simulink model "Hybrid2_article_SVC_stage1"  (R2025a)
settings: Solver=FixedStepAuto  StartTime=0.0  StopTime=0.2  FixedStep=Ts  RelTol=1e-3
undefined symbols (not defined in the file or in its folder): closedLoop, controller, D1, D11, Delta, DiscIntNeverNeededParam, find_system, grid, level, protection, sensor, solarPanel, solarPlant, Ts
libraries: powerlib_extras x38, nesl_utility x29, spsSampleandHoldLib x24, spsThyristorLib x24, spsSeriesRLCBranchLib x23, simulink x22, fl_lib x18, ee_lib x12, spsEdgeDetectorLib x12, spsParallelRLCBranchLib x10, spsThreePhaseVIMeasurementLib x9, simulink_extras x8
(part 5 of 8)

== system Hybrid2_article_SVC_stage1/Power Circuit/Power Circuit/Average ==
  note: Resistance is added for simulation purpose, as the solver need to resolve absolute voltage values
  m : Inport
  TripSig : Inport  Port=2
  Average-Value Voltage Source Converter : ee_lib/Semiconductors & Converters/Converters/Average-Value Voltage Source Converter (Three-Phase)  port_option=ee.enum.threePhasePort.composite  frequency_option=ee.enum.converters.frequency.variable  input_option=ee.enum.converters.inputOption.ModWave  FRated=60 Hz  losses_parameterization=ee.enum.converters.losses.fixed  Pfixed=1 W  ks=0.01  kc1=1.7 V  kc2=0.01 Ohm  Ploss_vect=[100, 800, 1870, 3250, 4900] W  Irms_vect=[10, 100, 200, 300, 400] A  Vdc_nom=300 V  thermal_mass=30000 J/K  temperature_specify=off  temperature_priority=High  temperature=298.15 K  temperature_nominal_specify=off  temperature_nominal_value=1  temperature_nominal_unit=K
      settings: InternalSimscapePortConfiguration="{\"Bottom\":[],\"Left\":[{\"id\":\"ModWave\",\"label\":\"ModWave\",\"type\":\"input\"},{\"id\":\"N\",\"label\":\"~\",\"type\":\"foundation.electrical.three_phase\"}],\"Right\":[{\"id\":\"p\",\"label\":\"+\",\"type\":\"foundation.electrical.electrical\"},{\"id\":\"n\",\"label\":\"-\",\"type\":\"foundation.electrical.electrical\"}],\"Top\":[]}"
  Electrical Reference : fl_lib/Electrical/Electrical Elements/Electrical Reference
  Open Circuit : fl_lib/Electrical/Electrical Elements/Open Circuit  v_specify=off  v_priority=None  v=0 V  v_nominal_specify=off  v_nominal_value=1  v_nominal_unit=V
  Resistor : fl_lib/Electrical/Electrical Elements/Resistor  R=1e6 Ohm  i_specify=off  i_priority=None  i=0 A  i_nominal_specify=off  i_nominal_value=1  i_nominal_unit=A  v_specify=off  v_priority=None  v=0 V  v_nominal_specify=off  v_nominal_value=1  v_nominal_unit=V
  Simulink-PS Converter6 : nesl_utility/Simulink-PS Converter  PhysicalDomain=network_engine_domain  SubClassName=ps_input  LeftPortType=input  RightPortType=output  PseudoPeriodic=off  Frequencies=[]  NoiseDistribution=none  NoiseParameters=[]  Unit=1  AffineConversion=off  FilteringAndDerivatives=provide  SimscapeFilterOrder=1  InputFilterTimeConstant=0.001  UdotUserProvided=0
  Terminator : Terminator
  + : PMIOPort  Side=Left
  - : PMIOPort  Port=2  Side=Left
  ABC : PMIOPort  Port=3  Side=Right
  O : PMIOPort  Port=4  Side=Left
  wires:
  TripSig/1 -> Terminator/1
  m/1 -> Simulink-PS Converter6/1
  connections:
  Average-Value Voltage Source Converter/LConn2 -- ABC/RConn1
  Average-Value Voltage Source Converter/LConn1 -- Simulink-PS Converter6/RConn1
  Average-Value Voltage Source Converter/RConn2 -- Resistor/LConn1 -- -/RConn1
  Average-Value Voltage Source Converter/RConn1 -- +/RConn1
  Open Circuit/LConn1 -- O/RConn1
  Resistor/RConn1 -- Electrical Reference/LConn1

== system Hybrid2_article_SVC_stage1/Power Circuit/Power Circuit/Three Level ==
  m : Inport
  TripSig : Inport  Port=2
  Gate : Subsystem
  Neutral point controller : slpidlib/PID Controller  Controller=P  Form=Parallel  TimeDomain=Discrete-time  UseExternalTs=off  SampleTime=-1  IntegratorMethod=Forward Euler  FilterMethod=Forward Euler  ControllerParametersSource=internal  P=0.001  I=80/2  UseKiTs=off  D=0  UseExternalDerivativeSource=off  N=100  UseFilter=on  TunerSelectOption=Transfer Function Based (PID Tuner App)  ZeroCross=off  InitialConditionSource=internal  InitialConditionForIntegrator=0  InitialConditionForFilter=0  DifferentiatorICPrevScaledInput=0  ExternalReset=none  TrackingMode=off  Kt=1  LimitOutput=on  SatLimitsSource=internal  UpperSaturationLimit=1  LowerSaturationLimit=-1  LinearizeAsGain=on  AntiWindupMode=back-calculation  Kb=1000  LimitIntegrator=off  UpperIntegratorSaturationLimit=inf  LowerIntegratorSaturationLimit=-inf  POutMin=[]  POutMax=[]  IOutMin=[]  IOutMax=[]  DOutMin=[]  DOutMax=[]  NOutMin=[]  NOutMax=[]  SumOutMin=[]  SumOutMax=[]  SaturationOutMin=[]  SaturationOutMax=[]  PParamMin=[]  PParamMax=[]  IParamMin=[]  IParamMax=[]  DParamMin=[]  DParamMax=[]  NParamMin=[]  NParamMax=[]  KbParamMin=[]  KbParamMax=[]  KtParamMin=[]  KtParamMax=[]  KbOutMin=[]  KbOutMax=[]  KtOutMin=[]  KtOutMax=[]  IntegratorOutMin=[]  IntegratorOutMax=[]  FilterOutMin=[]  FilterOutMax=[]  SumI1OutMin=[]  SumI1OutMax=[]  SumI2OutMin=[]  SumI2OutMax=[]  SumI3OutMin=[]  SumI3OutMax=[]  SumI4OutMin=[]  SumI4OutMax=[]  SumDOutMin=[]  SumDOutMax=[]  DifferentiatorOutMin=[]  DifferentiatorOutMax=[]  FilterDiffOutCoefMin=[]  FilterDiffOutCoefMax=[]  ReciprocalOutMin=[]  ReciprocalOutMax=[]  SumDenOutMin=[]  SumDenOutMax=[]  SumNumOutMin=[]  SumNumOutMax=[]  DivideOutMin=[]  DivideOutMax=[]  UdiffTsProdOutMin=[]  UdiffTsProdOutMax=[]  NTsProdOutMin=[]  NTsProdOutMax=[]  UintegralTsProdOutMin=[]  UintegralTsProdOutMax=[]  UngainTsProdOutMin=[]  UngainTsProdOutMax=[]  ClampingZeroOutDataTypeStr=Inherit: Inherit via back propagation  ClampingZeroOutMin=[]  ClampingZeroOutMax=[]  FilterDenConstantOutDataTypeStr=Inherit: Inherit via back propagation  FilterDenConstantOutMin=[]  FilterDenConstantOutMax=[]  PCopyOutDataTypeStr=Inherit: Inherit via back propagation  PCopyOutMin=[]  PCopyOutMax=[]  NCopyOutDataTypeStr=Inherit: Inherit via back propagation  NCopyOutMin=[]  NCopyOutMax=[]  IntegratorContinuousStateAttributes=''  IntegratorStateMustResolveToSignalObject=off  IntegratorRTWStateStorageClass=Auto  FilterContinuousStateAttributes=''  FilterStateMustResolveToSignalObject=off  FilterRTWStateStorageClass=Auto  ParallelPVariant=InternalParameters  IdealPVariant=Disabled  IVariant=Disabled  DVariant=Disabled  IntegratorVariant=Disabled  SatVariant=Enabled  AWVariant=Disabled  PCopyVariant=Disabled  TRVariant=Disabled  FdbkBlocksVariant=Forward  IdealPFdbkVariant=Disabled  SatFdbkVariant=Disabled  DerivativeFilterVariant=Disabled  NVariant=Disabled  NCopyVariant=Disabled_SignalSpec  FilterICVariant=Disabled  IntegratorICVariant=Disabled  ExternalResetVariant=Disabled  TRSumVariant=Passthrough  SumFdbkVariant=Disabled  SumVariant=Passthrough_P  TsampFilterVariant=InternalTs  TsampNgainVariant=Passthrough  TsampIntegralVariant=Disabled_SignalSpec  ExternalSaturationOutDataTypeStr=Inherit: Same as second input  DerivativeSourceVariant=Disabled  PreIntVariant=InternalPreInt
  "PWM Generator (Three-phase, Three-level)" : eePwmGeneratorThreeLevel/PWM Generator (Three-phase, Three-level)  CPWMMode=SPWM: sinusoidal PWM  fsw=solarPlant.switchFrequency  Ts=1/(10*solarPlant.switchFrequency)
      settings: SamplingMode=Natural
  Product : Product
  Product1 : Product
  Protection : Subsystem
  Sensing voltage Vc1 : Subsystem
      mask Display: disp('Vdc1')
  Sensing voltage Vc2 : Subsystem
      mask Display: disp('Vdc2')
  Step@1cycle : Step  Time=1/grid.frequency  SampleTime=1/(10*solarPlant.switchFrequency)
  Sum : Sum  Inputs=|+-
  Switch5 : Switch  Criteria=u2 > Threshold  Threshold=solarPlant.DCMPPTValue/2/2  SaturateOnIntegerOverflow=off  InputSameDT=off
  Terminator1 : Terminator
  Three-Level Converter (Three-Phase) : ee_lib/Semiconductors & Converters/Converters/Three-Level Converter (Three-Phase)  port_option=ee.enum.threePhasePort.composite  device_type=2  Vf=0.8 V  Ron=0.001 Ohm  Rds=0.001 Ohm  Goff=1e-6 1/Ohm  Vth=0.2 V  Vgt=1 V  Vgt_off=-1 V  Ih=1 A  K=0  diode_param=2  diode_Vf=0.8 V  diode_Ron=0.001 Ohm  diode_Goff=1e-5 1/Ohm  diode_C=50 nF  diode_iRM=-235 A  diode_iF=300 A  diode_idot=-50 A/us  diode_trr_param=1  diode_trr_factor=3  diode_trr=15 us  diode_Qrr=1500 s*uA  snubber_type=0  Cs=1e-7 F  Rs=0.1 Ohm
      settings: InternalSimscapePortConfiguration="{\"Bottom\":[],\"Left\":[{\"id\":\"G\",\"label\":\"G\",\"type\":\"foundation.electrical.twenty_four_phase\"},{\"id\":\"N\",\"label\":\"~\",\"type\":\"foundation.electrical.three_phase\"}],\"Right\":[{\"id\":\"p\",\"label\":\"+\",\"type\":\"foundation.electrical.electrical\"},{\"id\":\"z\",\"label\":\"0\",\"type\":\"foundation.electrical.electrical\"},{\"id\":\"n\",\"label\":\"-\",\"type\":\"foundation.electrical.electrical\"}],\"Top\":[]}"
  Zero-Order Hold1 : ZeroOrderHold  SampleTime=1/(10*solarPlant.switchFrequency)
  Zero-Order Hold2 : ZeroOrderHold  SampleTime=1/(5*solarPlant.switchFrequency)
  Zero-Order Hold3 : ZeroOrderHold  SampleTime=1/(5*solarPlant.switchFrequency)
  Zero-Order Hold4 : ZeroOrderHold  SampleTime=1/(10*solarPlant.switchFrequency)
  start MPPT Voltage : Constant  Value=solarPlant.DCMPPTValue/2
  + : PMIOPort  Side=Left
  - : PMIOPort  Port=2  Side=Left
  ABC : PMIOPort  Port=3  Side=Right
  O : PMIOPort  Port=4  Side=Left
  wires:
  Sum/1 -> Neutral point controller/1
  Switch5/1 -> Zero-Order Hold4/1, Product1/2
  m/1 -> Product1/1
  Zero-Order Hold2/1 -> Sum/1
  [Vpv] -> Switch5/2, Switch5/1
  Protection/1(PWM) -> Gate/1(g)
  Zero-Order Hold3/1 -> Sum/2
  "PWM Generator (Three-phase, Three-level)"/1 -> Protection/2(G)
  Zero-Order Hold1/1 -> "PWM Generator (Three-phase, Three-level)"/1
  Zero-Order Hold4/1 -> "PWM Generator (Three-phase, Three-level)"/2
  "PWM Generator (Three-phase, Three-level)"/2 -> Terminator1/1
  Product1/1 -> Zero-Order Hold1/1
  [Vdc1] -> Zero-Order Hold2/1
  start MPPT Voltage/1 -> Switch5/3
  TripSig/1 -> Protection/1(TripSig)
  Step@1cycle/1 -> Product/2
  [Vdc2] -> Zero-Order Hold3/1
  Neutral point controller/1 -> Product/1
  Product/1 -> "PWM Generator (Three-phase, Three-level)"/3
  connections:
  Three-Level Converter (Three-Phase)/RConn2 -- O/RConn1 -- Sensing voltage Vc2/LConn1 -- Sensing voltage Vc1/RConn1
  Three-Level Converter (Three-Phase)/RConn3 -- -/RConn1 -- Sensing voltage Vc2/RConn1
  Three-Level Converter (Three-Phase)/RConn1 -- +/RConn1 -- Sensing voltage Vc1/LConn1
  Three-Level Converter (Three-Phase)/LConn2 -- ABC/RConn1
  Gate/RConn1 -- Three-Level Converter (Three-Phase)/LConn1

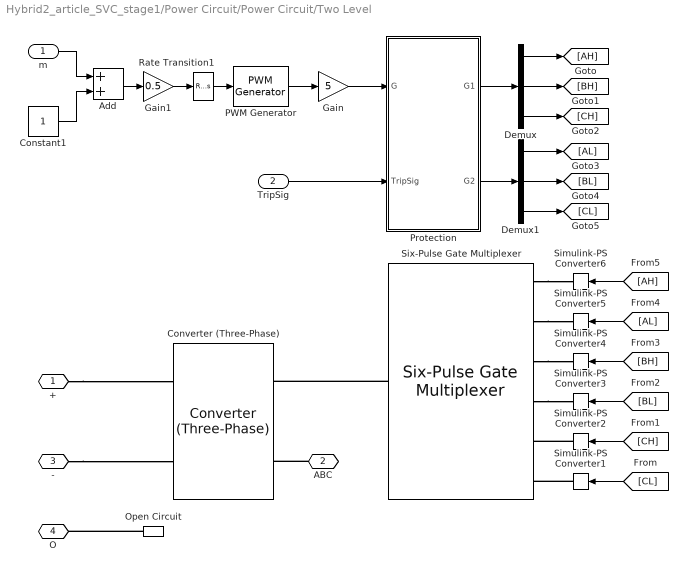
== system Hybrid2_article_SVC_stage1/Power Circuit/Power Circuit/Two Level ==
  m : Inport
  TripSig : Inport  Port=2
  Add : Sum
  Constant1 : Constant
  Converter (Three-Phase) : ee_lib/Semiconductors & Converters/Converters/Converter (Three-Phase)  port_option=ee.enum.threePhasePort.composite  fidelity_option=ee.enum.converters.fidelity.detailed  device_type=ee.enum.converters.switchingdevice.ideal  showThermalPort=false  K=0  Vth=0.5 V  Vgt=1 V  Vgt_off=-1 V  Ih=1 A  Vf=0.8 V  Ron=0.001 Ohm  Rds=0.001 Ohm  Goff=1e-6 1/Ohm  Eon_scalar=22.86e-3 J  Eoff_scalar=17.14e-3 J  Eoff_natural_commutation=10e-3 J  Voff=300 V  Iout_scalar=600 A  onCurrentMeasDelay=0 s  useCurrentFromPreviousCycle=false  useVoltageFromPreviousCycle=false  diode_param=ee.enum.converters.protectiondiode.nodynamics  diode_Vf=0.01 V  diode_Ron=0.0001 Ohm  diode_Goff=1e-5 1/Ohm  diode_C=50 nF  diode_iRM=-235 A  diode_iF=300 A  diode_idot=-50 A/us  diode_trr_param=ee.enum.converters.diodetrr.trr_factor  diode_trr_factor=3  diode_trr=15 us  diode_Qrr=1500 s*uA  diode_rec_loss_model=ee.enum.diode.reverseRecoveryModel.fixed  diode_ErecVal=0 J  diode_scaleWithIandV=false  diode_ErecMat=zeros(2, 3) J  diode_TjrecVec=[298.15, 398.15] K  diode_IfrecVec=[.1, 1, 10] A  diode_IrecVal=10 A  diode_VrecVal=10 V  diode_tFilter=1 / 1000 / 100 s  thermal_network_parameterization=ee.enum.thermalNetworkTopology.external  Rth=[.08, .5] K/W  Rth_Cauer=[.08, .1, .5] K/W  Rth_Foster=[.08, .14, .22, .16] K/W  thermal_mass_parameterization=ee.enum.thermalNetwork.timeconstant  thermal_mass=[.01, .5] J/K  thermal_mass_Cauer=[.01, .1, .5] J/K  thermal_mass_Foster=[.001, .005, .05, .5] J/K  thermal_time_constant=[.001, .2] s  thermal_time_constant_Cauer=[.001, .1, .2] s  thermal_time_constant_Foster=[7e-05, .0007, .01, .08] s  thermal_mass_initial_temperatures=[25, 25] degC  thermal_mass_initial_temperatures_Cauer=[25, 25, 25] degC  junction_thermal_mass=0.01 J/K  Tvec_initial_Foster=[25, 25, 25, 25] degC  snubber_type=ee.enum.converters.snubber.exclude  Cs=1e-7 F  Rs=0.1 Ohm  Vce_loss=[0, 150, 300] V
  Demux : Demux  Outputs=3
  Demux1 : Demux  Outputs=3
  Gain : Gain  Gain=5
  Gain1 : Gain  Gain=0.5
  Open Circuit : fl_lib/Electrical/Electrical Elements/Open Circuit  v_specify=off  v_priority=None  v=0 V  v_nominal_specify=off  v_nominal_value=1  v_nominal_unit=V
  PWM Generator : eePwmGenerator/PWM Generator  CarrCount=Up  Tper=1/solarPlant.switchFrequency  Tdelay=0  Ts=1/(10*solarPlant.switchFrequency)
  Protection : Subsystem
  Rate Transition1 : RateTransition  OutPortSampleTime=1/(10*solarPlant.switchFrequency)
  Simulink-PS Converter{1..6} (6 alike) : nesl_utility/Simulink-PS Converter  PhysicalDomain=network_engine_domain  SubClassName=ps_input  LeftPortType=input  RightPortType=output  PseudoPeriodic=off  Frequencies=[]  NoiseDistribution=none  NoiseParameters=[]  Unit=1  AffineConversion=off  FilteringAndDerivatives=provide  SimscapeFilterOrder=1  InputFilterTimeConstant=0.001  UdotUserProvided=0
  Six-Pulse Gate Multiplexer : ee_lib/Semiconductors & Converters/Converters/Six-Pulse Gate Multiplexer  port_option=ee.enum.controlport.ps
  + : PMIOPort  Side=Left
  ABC : PMIOPort  Port=2  Side=Right
  - : PMIOPort  Port=3  Side=Left
  O : PMIOPort  Port=4  Side=Left
  wires:
  Rate Transition1/1 -> PWM Generator/1
  [CL] -> Simulink-PS Converter1/1
  [AH] -> Simulink-PS Converter6/1
  Demux1/3 -> [CL]
  m/1 -> Add/1
  [CH] -> Simulink-PS Converter2/1
  Demux/2 -> [BH]
  Demux1/2 -> [BL]
  Demux/3 -> [CH]
  TripSig/1 -> Protection/2(TripSig)
  Demux1/1 -> [AL]
  [BH] -> Simulink-PS Converter4/1
  Protection/2(G2) -> Demux1/1
  Protection/1(G1) -> Demux/1
  PWM Generator/1 -> Gain/1
  [AL] -> Simulink-PS Converter5/1
  [BL] -> Simulink-PS Converter3/1
  Constant1/1 -> Add/2
  Gain/1 -> Protection/1(G)
  Add/1 -> Gain1/1
  Gain1/1 -> Rate Transition1/1
  Demux/1 -> [AH]
  connections:
  Open Circuit/LConn1 -- O/RConn1
  Simulink-PS Converter2/RConn1 -- Six-Pulse Gate Multiplexer/LConn5
  ABC/RConn1 -- Converter (Three-Phase)/LConn2
  Six-Pulse Gate Multiplexer/RConn1 -- Converter (Three-Phase)/LConn1
  Six-Pulse Gate Multiplexer/LConn2 -- Simulink-PS Converter5/RConn1
  +/RConn1 -- Converter (Three-Phase)/RConn1
  -/RConn1 -- Converter (Three-Phase)/RConn2
  Six-Pulse Gate Multiplexer/LConn4 -- Simulink-PS Converter3/RConn1
  Six-Pulse Gate Multiplexer/LConn3 -- Simulink-PS Converter4/RConn1
  Six-Pulse Gate Multiplexer/LConn1 -- Simulink-PS Converter6/RConn1
  Simulink-PS Converter1/RConn1 -- Six-Pulse Gate Multiplexer/LConn6

== system Hybrid2_article_SVC_stage1/SVC Controller1/Firing Unit/Firing Unit AB ==
  note: PLL
      | sync on
      | pos. peak
      | of input
  note: Generate firing
      | pulses for TSC3
  note: Generate firing
      | pulse for TCR +
  note: Generate firing
      | pulse for TCR -
  note: Generate firing
      | pulses for TSC2
  note: Generate firing
      | pulses for TSC1
  note: Generate square-wave lagging Input
      | voltage by 90 degrees and pulses (width of
      | one sample) for positive (Sync +)
      | and negative (Sync -) transition
  note: Compute number
      | of samples per cycle
  note: Input
      | voltage
  V : Inport  PortDimensions=1
  Alpha : Inport  Port=2  PortDimensions=1
  TSC1_On : Inport  Port=3  PortDimensions=1
  TSC2_On : Inport  Port=4  PortDimensions=1
  TSC3_On : Inport  Port=5  PortDimensions=1
  BL2 : Subsystem
  BL3 : Subsystem
  Correction for delay : Gain  Gain=Nstep*Ts*2*pi  SaturateOnIntegerOverflow=on  OutDataTypeStr=Inherit: Same as input  ParamDataTypeStr=Inherit: Same as input
  Logical Operator2 : Logic  Operator=NOT  Inputs=3
  "PLL sync on positive peak " : Subsystem  mask(Discrete 1-phase PLL){Par_Init=[PhaseInit FreqInit], ParK=[120 2800], Ts=Ts}
      mask prompts: Par_Init "Initial input:[ Phase(degrees)   Frequency(Hz) ]"; ParK "Regulator gains [ Kp  Ki ]"; Ts "Sample time:"
      mask help:
      | This Phase Locked Loop (PLL) system can be used  to synchronize on a variable frequency sinusoidal signal.
      |
      | Input 1: Normalized input signal V(pu)
      mask init:
      | Kp=ParK(1);
      | Ki=ParK(2);
      | Phase_Init=Par_Init(1);
      | Finit=Par_Init(2);
  Sum : Sum  InputSameDT=on  SaturateOnIntegerOverflow=on  OutDataTypeStr=Inherit: Same as first input
  TCR Pulse Generatorr : Subsystem
  TCR Pulse Generatorr1 : Subsystem  mask{Ts=Ts}
      mask prompts: Ts "Sample time:"
  TCS Pulse Generator : Subsystem
  TCS Pulse Generator1 : Subsystem
  TCS Pulse Generator2 : Subsystem
  Trigonometric Function6 : Trigonometry
  TCR + : Outport  VectorParamsAs1DForOutWhenUnconnected=off
  TCR - : Outport  Port=2  VectorParamsAs1DForOutWhenUnconnected=off
  TSC1 + : Outport  Port=3  VectorParamsAs1DForOutWhenUnconnected=off
  TSC1 - : Outport  Port=4  VectorParamsAs1DForOutWhenUnconnected=off
  TSC2 + : Outport  Port=5  VectorParamsAs1DForOutWhenUnconnected=off
  TSC2 - : Outport  Port=6  VectorParamsAs1DForOutWhenUnconnected=off
  TSC3 + : Outport  Port=7  VectorParamsAs1DForOutWhenUnconnected=off
  TSC3 - : Outport  Port=8  VectorParamsAs1DForOutWhenUnconnected=off
  wires:
  Logical Operator2/1 -> TCR Pulse Generatorr1/4(SqWave)
  TCR Pulse Generatorr/1(TCR +/-) -> TCR +/1
  BL3/1(SqWave) -> TCS Pulse Generator/1(SqWave), TCS Pulse Generator2/1(SqWave), TCS Pulse Generator1/1(SqWave), TCR Pulse Generatorr/4(SqWave), Logical Operator2/1
  TCS Pulse Generator2/2(TSC -) -> TSC3 -/1
  TCS Pulse Generator2/1(TSC +) -> TSC3 +/1
  TSC3_On/1 -> TCS Pulse Generator2/4(TSC_On)
  TCR Pulse Generatorr1/1(TCR +/-) -> TCR -/1
  TCS Pulse Generator/2(TSC -) -> TSC1 -/1
  TCS Pulse Generator/1(TSC +) -> TSC1 +/1
  BL3/2(Sync +) -> TCS Pulse Generator2/2(Sync +), TCS Pulse Generator1/2(Sync +), TCS Pulse Generator/2(Sync +), TCR Pulse Generatorr/3(Sync +/-)
  BL3/3(Sync -) -> TCS Pulse Generator/3(Sync -), TCS Pulse Generator2/3(Sync -), TCS Pulse Generator1/3(Sync -), TCR Pulse Generatorr1/3(Sync +/-)
  Alpha/1 -> TCR Pulse Generatorr/2(Alpha), TCR Pulse Generatorr1/2(Alpha)
  TSC1_On/1 -> TCS Pulse Generator/4(TSC_On)
  TCS Pulse Generator1/2(TSC -) -> TSC2 -/1
  TCS Pulse Generator1/1(TSC +) -> TSC2 +/1
  TSC2_On/1 -> TCS Pulse Generator1/4(TSC_On)
  BL2/1(Ns/c) -> TCR Pulse Generatorr/1(Ns/c), TCR Pulse Generatorr1/1(Ns/c)
  "PLL sync on positive peak "/2(wt) -> Sum/2
  Sum/1 -> Trigonometric Function6/1
  Trigonometric Function6/1 -> BL3/2(sin(wt))
  Correction for delay/1 -> Sum/1
  "PLL sync on positive peak "/1(Freq) -> BL2/1(Freq), BL3/1(Freq), Correction for delay/1
  V/1 -> "PLL sync on positive peak "/1(V(pu))

== system Hybrid2_article_SVC_stage1/SVC Controller1/Firing Unit/Firing Unit BC ==
  note: PLL
      | sync on
      | pos. peak
      | of input
  note: Generate firing
      | pulses for TSC3
  note: Generate firing
      | pulse for TCR +
  note: Generate firing
      | pulse for TCR -
  note: Generate firing
      | pulses for TSC2
  note: Generate firing
      | pulses for TSC1
  note: Generate square-wave lagging Input
      | voltage by 90 degrees and pulses (width of
      | one sample) for positive (Sync +)
      | and negative (Sync -) transition
  note: Compute number
      | of samples per cycle
  note: Input
      | voltage
  V : Inport  PortDimensions=1
  Alpha : Inport  Port=2  PortDimensions=1
  TSC1_On : Inport  Port=3  PortDimensions=1
  TSC2_On : Inport  Port=4  PortDimensions=1
  TSC3_On : Inport  Port=5  PortDimensions=1
  BL2 : Subsystem
  BL3 : Subsystem
  Correction for delay : Gain  Gain=Nstep*Ts*2*pi  SaturateOnIntegerOverflow=on  OutDataTypeStr=Inherit: Same as input  ParamDataTypeStr=Inherit: Same as input
  Logical Operator2 : Logic  Operator=NOT  Inputs=3
  "PLL sync on positive peak " : Subsystem  mask(Discrete 1-phase PLL){Par_Init=[PhaseInit FreqInit], ParK=[120 2800], Ts=Ts}
      mask prompts: Par_Init "Initial input:[ Phase(degrees)   Frequency(Hz) ]"; ParK "Regulator gains [ Kp  Ki ]"; Ts "Sample time:"
      mask help:
      | This Phase Locked Loop (PLL) system can be used  to synchronize on a variable frequency sinusoidal signal.
      |
      | Input 1: Normalized input signal V(pu)
      mask init:
      | Kp=ParK(1);
      | Ki=ParK(2);
      | Phase_Init=Par_Init(1);
      | Finit=Par_Init(2);
  Sum : Sum  InputSameDT=on  SaturateOnIntegerOverflow=on  OutDataTypeStr=Inherit: Same as first input
  TCR Pulse Generatorr : Subsystem  mask{Ts=Ts}
      mask prompts: Ts "Sample time:"
  TCR Pulse Generatorr1 : Subsystem  mask{Ts=Ts}
      mask prompts: Ts "Sample time:"
  TCS Pulse Generator : Subsystem
  TCS Pulse Generator1 : Subsystem
  TCS Pulse Generator2 : Subsystem
  Trigonometric Function6 : Trigonometry
  TCR + : Outport  VectorParamsAs1DForOutWhenUnconnected=off
  TCR - : Outport  Port=2  VectorParamsAs1DForOutWhenUnconnected=off
  TSC1 + : Outport  Port=3  VectorParamsAs1DForOutWhenUnconnected=off
  TSC1 - : Outport  Port=4  VectorParamsAs1DForOutWhenUnconnected=off
  TSC2 + : Outport  Port=5  VectorParamsAs1DForOutWhenUnconnected=off
  TSC2 - : Outport  Port=6  VectorParamsAs1DForOutWhenUnconnected=off
  TSC3 + : Outport  Port=7  VectorParamsAs1DForOutWhenUnconnected=off
  TSC3 - : Outport  Port=8  VectorParamsAs1DForOutWhenUnconnected=off
  wires:
  Logical Operator2/1 -> TCR Pulse Generatorr1/4(SqWave)
  TCR Pulse Generatorr/1(TCR +/-) -> TCR +/1
  BL3/1(SqWave) -> TCS Pulse Generator/1(SqWave), TCS Pulse Generator2/1(SqWave), TCS Pulse Generator1/1(SqWave), TCR Pulse Generatorr/4(SqWave), Logical Operator2/1
  TCS Pulse Generator2/2(TSC -) -> TSC3 -/1
  TCS Pulse Generator2/1(TSC +) -> TSC3 +/1
  TSC3_On/1 -> TCS Pulse Generator2/4(TSC_On)
  TCR Pulse Generatorr1/1(TCR +/-) -> TCR -/1
  TCS Pulse Generator/2(TSC -) -> TSC1 -/1
  TCS Pulse Generator/1(TSC +) -> TSC1 +/1
  BL3/2(Sync +) -> TCS Pulse Generator2/2(Sync +), TCS Pulse Generator1/2(Sync +), TCS Pulse Generator/2(Sync +), TCR Pulse Generatorr/3(Sync +/-)
  BL3/3(Sync -) -> TCS Pulse Generator/3(Sync -), TCS Pulse Generator2/3(Sync -), TCS Pulse Generator1/3(Sync -), TCR Pulse Generatorr1/3(Sync +/-)
  Alpha/1 -> TCR Pulse Generatorr/2(Alpha), TCR Pulse Generatorr1/2(Alpha)
  TSC1_On/1 -> TCS Pulse Generator/4(TSC_On)
  TCS Pulse Generator1/2(TSC -) -> TSC2 -/1
  TCS Pulse Generator1/1(TSC +) -> TSC2 +/1
  TSC2_On/1 -> TCS Pulse Generator1/4(TSC_On)
  BL2/1(Ns/c) -> TCR Pulse Generatorr/1(Ns/c), TCR Pulse Generatorr1/1(Ns/c)
  "PLL sync on positive peak "/2(wt) -> Sum/2
  Sum/1 -> Trigonometric Function6/1
  Trigonometric Function6/1 -> BL3/2(sin(wt))
  Correction for delay/1 -> Sum/1
  "PLL sync on positive peak "/1(Freq) -> BL2/1(Freq), BL3/1(Freq), Correction for delay/1
  V/1 -> "PLL sync on positive peak "/1(V(pu))

== system Hybrid2_article_SVC_stage1/SVC Controller1/Firing Unit/Firing Unit CA ==
  note: PLL
      | sync on
      | pos. peak
      | of input
  note: Generate firing
      | pulses for TSC3
  note: Generate firing
      | pulse for TCR +
  note: Generate firing
      | pulse for TCR -
  note: Generate firing
      | pulses for TSC2
  note: Generate firing
      | pulses for TSC1
  note: Generate square-wave lagging Input
      | voltage by 90 degrees and pulses (width of
      | one sample) for positive (Sync +)
      | and negative (Sync -) transition
  note: Compute number
      | of samples per cycle
  note: Input
      | voltage
  V : Inport  PortDimensions=1
  Alpha : Inport  Port=2  PortDimensions=1
  TSC1_On : Inport  Port=3  PortDimensions=1
  TSC2_On : Inport  Port=4  PortDimensions=1
  TSC3_On : Inport  Port=5  PortDimensions=1
  BL2 : Subsystem
  BL3 : Subsystem
  Correction for delay : Gain  Gain=Nstep*Ts*2*pi  SaturateOnIntegerOverflow=on  OutDataTypeStr=Inherit: Same as input  ParamDataTypeStr=Inherit: Same as input
  Logical Operator2 : Logic  Operator=NOT  Inputs=3
  "PLL sync on positive peak " : Subsystem  mask(Discrete 1-phase PLL){Par_Init=[PhaseInit FreqInit], ParK=[120 2800], Ts=Ts}
      mask prompts: Par_Init "Initial input:[ Phase(degrees)   Frequency(Hz) ]"; ParK "Regulator gains [ Kp  Ki ]"; Ts "Sample time:"
      mask help:
      | This Phase Locked Loop (PLL) system can be used  to synchronize on a variable frequency sinusoidal signal.
      |
      | Input 1: Normalized input signal V(pu)
      mask init:
      | Kp=ParK(1);
      | Ki=ParK(2);
      | Phase_Init=Par_Init(1);
      | Finit=Par_Init(2);
  Sum : Sum  InputSameDT=on  SaturateOnIntegerOverflow=on  OutDataTypeStr=Inherit: Same as first input
  TCR Pulse Generatorr : Subsystem  mask{Ts=Ts}
      mask prompts: Ts "Sample time:"
  TCR Pulse Generatorr1 : Subsystem  mask{Ts=Ts}
      mask prompts: Ts "Sample time:"
  TCS Pulse Generator : Subsystem
  TCS Pulse Generator1 : Subsystem
  TCS Pulse Generator2 : Subsystem
  Trigonometric Function6 : Trigonometry
  TCR + : Outport  VectorParamsAs1DForOutWhenUnconnected=off
  TCR - : Outport  Port=2  VectorParamsAs1DForOutWhenUnconnected=off
  TSC1 + : Outport  Port=3  VectorParamsAs1DForOutWhenUnconnected=off
  TSC1 - : Outport  Port=4  VectorParamsAs1DForOutWhenUnconnected=off
  TSC2 + : Outport  Port=5  VectorParamsAs1DForOutWhenUnconnected=off
  TSC2 - : Outport  Port=6  VectorParamsAs1DForOutWhenUnconnected=off
  TSC3 + : Outport  Port=7  VectorParamsAs1DForOutWhenUnconnected=off
  TSC3 - : Outport  Port=8  VectorParamsAs1DForOutWhenUnconnected=off
  wires:
  Logical Operator2/1 -> TCR Pulse Generatorr1/4(SqWave)
  TCR Pulse Generatorr/1(TCR +/-) -> TCR +/1
  BL3/1(SqWave) -> TCS Pulse Generator/1(SqWave), TCS Pulse Generator2/1(SqWave), TCS Pulse Generator1/1(SqWave), TCR Pulse Generatorr/4(SqWave), Logical Operator2/1
  TCS Pulse Generator2/2(TSC -) -> TSC3 -/1
  TCS Pulse Generator2/1(TSC +) -> TSC3 +/1
  TSC3_On/1 -> TCS Pulse Generator2/4(TSC_On)
  TCR Pulse Generatorr1/1(TCR +/-) -> TCR -/1
  TCS Pulse Generator/2(TSC -) -> TSC1 -/1
  TCS Pulse Generator/1(TSC +) -> TSC1 +/1
  BL3/2(Sync +) -> TCS Pulse Generator2/2(Sync +), TCS Pulse Generator1/2(Sync +), TCS Pulse Generator/2(Sync +), TCR Pulse Generatorr/3(Sync +/-)
  BL3/3(Sync -) -> TCS Pulse Generator/3(Sync -), TCS Pulse Generator2/3(Sync -), TCS Pulse Generator1/3(Sync -), TCR Pulse Generatorr1/3(Sync +/-)
  Alpha/1 -> TCR Pulse Generatorr/2(Alpha), TCR Pulse Generatorr1/2(Alpha)
  TSC1_On/1 -> TCS Pulse Generator/4(TSC_On)
  TCS Pulse Generator1/2(TSC -) -> TSC2 -/1
  TCS Pulse Generator1/1(TSC +) -> TSC2 +/1
  TSC2_On/1 -> TCS Pulse Generator1/4(TSC_On)
  BL2/1(Ns/c) -> TCR Pulse Generatorr/1(Ns/c), TCR Pulse Generatorr1/1(Ns/c)
  "PLL sync on positive peak "/2(wt) -> Sum/2
  Sum/1 -> Trigonometric Function6/1
  Trigonometric Function6/1 -> BL3/2(sin(wt))
  Correction for delay/1 -> Sum/1
  "PLL sync on positive peak "/1(Freq) -> BL2/1(Freq), BL3/1(Freq), Correction for delay/1
  V/1 -> "PLL sync on positive peak "/1(V(pu))

== system Hybrid2_article_SVC_stage1/DFIG Wind Turbine/Control/Measurement and Transformation/ Improved Discrete 3-phase PLL ==
  note: Pierre Giroux, Gilbert Sybille, R. Gagnon
      | Power System Laboratory, IREQ
      | Hydro-Quebec
  note: New Discrete 3-phase PLL
  Vabc_pu : Inport  PortDimensions=3
  2nd-Order Filter : powerlib_extras/Discrete  Control Blocks/Discrete  2nd-Order Filter  FilterType=Lowpass  Fo=25  Zeta=0.707  Ts=Ts  Initialize=on  Vac_Init=[0 0 Finit]  Vdc_Init=Finit  PlotResponse=off  param1=[1 500 0.1]
  Constant1 : Constant  Value=2*pi*Finit
  Constant4 : Constant  Value=2*pi
  Discrete-Time Integrator : DiscreteIntegrator  SampleTime=Ts  ICPrevOutput=DiscIntNeverNeededParam  ICPrevScaledInput=DiscIntNeverNeededParam
  Discrete-Time Integrator1 : DiscreteIntegrator  gainval=1  SampleTime=Ts  LimitOutput=on  UpperSaturationLimit=2*pi*5  LowerSaturationLimit=-2*pi*5  ICPrevOutput=DiscIntNeverNeededParam  ICPrevScaledInput=DiscIntNeverNeededParam
  Gain10 : Gain  Gain=1/2/pi  SaturateOnIntegerOverflow=on  OutDataTypeStr=Inherit: Same as input  ParamDataTypeStr=Inherit: Same as input
  Kp1 : Gain  Gain=Kp2  SaturateOnIntegerOverflow=on  OutDataTypeStr=Inherit: Same as input  ParamDataTypeStr=Inherit: Same as input
  Kp2 : Gain  Gain=Ki2  SaturateOnIntegerOverflow=on  OutDataTypeStr=Inherit: Same as input  ParamDataTypeStr=Inherit: Same as input
  Kp3 : Gain  Gain=Ki1  SaturateOnIntegerOverflow=on  OutDataTypeStr=Inherit: Same as input  ParamDataTypeStr=Inherit: Same as input
  Kp4 : Gain  Gain=Kp1  SaturateOnIntegerOverflow=on  OutDataTypeStr=Inherit: Same as input  ParamDataTypeStr=Inherit: Same as input
  Math Function : Math  Operator=mod  SignedPower=on
  Mux2 : Mux  Inputs=2
  Rate Limiter : powerlib_extras/Discrete  Control Blocks/Discrete Rate Limiter  R=12  F=-12  Vinit=Finit  Ts=Ts
  Selector : Selector  InputPortWidth=3  IndexOptions=Index vector (dialog)  Indices=2  OutputSizes=1
  Sum : Sum  Inputs=+++
  Trigonometric Function : Trigonometry
  Trigonometric Function1 : Trigonometry  Operator=atan
  Trigonometric Function2 : Trigonometry  Operator=cos
  Trigonometric Function3 : Trigonometry  Operator=atan
  Unit Delay : UnitDelay  InitialCondition=Finit  SampleTime=Ts  HasFrameUpgradeWarning=on
  Variable Frequency Mean value : powerlib_extras/Discrete Measurements/Discrete Variable Frequency Mean value  Finit=Finit  Fmin=Fmin  Vinit=0  Ts=Ts
  abc_to_dq0 Transformation : powerlib_extras/Measurements/abc_to_dq0 Transformation
  Freq_Hz : Outport  VectorParamsAs1DForOutWhenUnconnected=off
  wt_rad : Outport  Port=2  VectorParamsAs1DForOutWhenUnconnected=off
  Sin_Cos : Outport  Port=3  VectorParamsAs1DForOutWhenUnconnected=off
  wires:
  Discrete-Time Integrator1/1 -> Sum/2
  Kp1/1 -> Sum/1
  Discrete-Time Integrator/1 -> Math Function/1
  Unit Delay/1 -> Variable Frequency Mean value/1, Freq_Hz/1
  Sum/1 -> Gain10/1, Discrete-Time Integrator/1
  Kp2/1 -> Discrete-Time Integrator1/1
  Trigonometric Function3/1 -> Kp2/1
  Kp3/1 -> Trigonometric Function3/1
  Variable Frequency Mean value/1 -> Kp3/1, Kp4/1
  Constant1/1 -> Sum/3
  Trigonometric Function1/1 -> Kp1/1
  Kp4/1 -> Trigonometric Function1/1
  Selector/1 -> Variable Frequency Mean value/2  "Vq"
  2nd-Order Filter/1 -> Unit Delay/1
  Rate Limiter/1 -> 2nd-Order Filter/1
  Gain10/1 -> Rate Limiter/1
  Mux2/1 -> abc_to_dq0 Transformation/2, Sin_Cos/1
  Trigonometric Function2/1 -> Mux2/2
  Trigonometric Function/1 -> Mux2/1
  Math Function/1 -> wt_rad/1, Trigonometric Function2/1, Trigonometric Function/1
  Constant4/1 -> Math Function/2
  abc_to_dq0 Transformation/1 -> Selector/1
  Vabc_pu/1 -> abc_to_dq0 Transformation/1

== system Hybrid2_article_SVC_stage1/DFIG Wind Turbine/Control/Measurement and Transformation/Discrete 3-phase PLL-Driven Positive-Sequence Active & Reactive Power ==
  note: Discrete 3-phase PLL-driven Positive-Sequence Active & Reactive Power
  note: Pierre Giroux, Gilbert Sybille
      | Power System Simulation Laboratory
      | IREQ, Hydro-Quebc
  Freq_Hz : Inport  PortDimensions=1
  Sin_Cos : Inport  Port=2  PortDimensions=2
  Vabc_V : Inport  Port=3  PortDimensions=3
  Iabc_A : Inport  Port=4  PortDimensions=3
  Deg->Rad : Gain  Gain=pi/180  SaturateOnIntegerOverflow=on  OutDataTypeStr=Inherit: Same as input  ParamDataTypeStr=Inherit: Same as input
  Discrete 3-phase PLL-Driven Positive-Sequence Fundamental Value : Subsystem  mask(Discrete 3-phase PLL-Driven Positive-Sequence Fundamental Value){Finit=Finit, Fmin=Fmin, Par_Init=Par_Vinit, Ts=Ts}
      mask prompts: Finit "Initial frequency (Hz):"; Fmin "Minimum frequency (Hz):"; Par_Init "Initial input (positive component): [ Mag  Phase-relative-to-PLL(degrees) ]"; Ts "Sample time:"
      mask help:
      | For a supplied fundamental frequency (port Freq), this discrete block computes  the positive-sequence component (Magnitude and Phase)  of a set of three balanced or unbalanced signals (port abc) which may contain harmonics.
      |  Input port "Sin_Cos" (a two-dimension signal) provides the reference frame required for the computation..
      |  First and second outputs return respectively the magnitude and phase (in degrees relative to the PLL phase)) of the fundamental.
      | For the first cycle of simulation, the outputs are held constant to the values specified by the parameter "Initial input".
      | constant to the values specified by the parameter "Initial input". The value of the parameter "Minimum frequency" is used to determine the buffer size of the "Variable Transport Delay" block found inside this subsystem.
      mask init:
      | Real_Init=Par_Init(1)*cos(pi/180*Par_Init(2));
      | Imag_Init=Par_Init(1)*sin(pi/180*Par_Init(2));
      | power_initmask();
      settings: OpenFcn=power_openblockproxy();
  Discrete 3-phase PLL-Driven Positive-Sequence Fundamental Value2 : Subsystem  mask(Discrete 3-phase PLL-Driven Positive-Sequence Fundamental Value){Finit=Finit, Fmin=Fmin, Par_Init=Par_Iinit, Ts=Ts}
      mask prompts: Finit "Initial frequency (Hz):"; Fmin "Minimum frequency (Hz):"; Par_Init "Initial input (positive component): [ Mag  Phase-relative-to-PLL(degrees) ]"; Ts "Sample time:"
      mask help:
      | For a supplied fundamental frequency (port Freq), this discrete block computes  the positive-sequence component (Magnitude and Phase)  of a set of three balanced or unbalanced signals (port abc) which may contain harmonics.
      |  Input port "Sin_Cos" (a two-dimension signal) provides the reference frame required for the computation..
      |  First and second outputs return respectively the magnitude and phase (in degrees relative to the PLL phase)) of the fundamental.
      | For the first cycle of simulation, the outputs are held constant to the values specified by the parameter "Initial input".
      | constant to the values specified by the parameter "Initial input". The value of the parameter "Minimum frequency" is used to determine the buffer size of the "Variable Transport Delay" block found inside this subsystem.
      mask init:
      | Real_Init=Par_Init(1)*cos(pi/180*Par_Init(2));
      | Imag_Init=Par_Init(1)*sin(pi/180*Par_Init(2));
      | power_initmask();
      settings: OpenFcn=power_openblockproxy();
  Gain1 : Gain  Gain=3/2  SaturateOnIntegerOverflow=on  OutDataTypeStr=Inherit: Same as input  ParamDataTypeStr=Inherit: Same as input
  Gain2 : Gain  Gain=3/2  SaturateOnIntegerOverflow=on  OutDataTypeStr=Inherit: Same as input  ParamDataTypeStr=Inherit: Same as input
  Product : Product  InputSameDT=on  SaturateOnIntegerOverflow=on  OutDataTypeStr=Inherit: Same as first input
  Product1 : Product  InputSameDT=on  SaturateOnIntegerOverflow=on  OutDataTypeStr=Inherit: Same as first input
  Product2 : Product  InputSameDT=on  SaturateOnIntegerOverflow=on  OutDataTypeStr=Inherit: Same as first input
  Sum : Sum  Inputs=+-  InputSameDT=on  SaturateOnIntegerOverflow=on  OutDataTypeStr=Inherit: Same as first input
  Trigonometric Function : Trigonometry
  Trigonometric Function1 : Trigonometry  Operator=cos
  Mag_V_V : Outport  VectorParamsAs1DForOutWhenUnconnected=off
  P_W : Outport  Port=2  VectorParamsAs1DForOutWhenUnconnected=off
  Q_Var : Outport  Port=3  VectorParamsAs1DForOutWhenUnconnected=off
  wires:
  Vabc_V/1 -> Discrete 3-phase PLL-Driven Positive-Sequence Fundamental Value/3(abc)
  Freq_Hz/1 -> Discrete 3-phase PLL-Driven Positive-Sequence Fundamental Value/1(Freq), Discrete 3-phase PLL-Driven Positive-Sequence Fundamental Value2/1(Freq)
  Sin_Cos/1 -> Discrete 3-phase PLL-Driven Positive-Sequence Fundamental Value/2(Sin_Cos), Discrete 3-phase PLL-Driven Positive-Sequence Fundamental Value2/2(Sin_Cos)
  Discrete 3-phase PLL-Driven Positive-Sequence Fundamental Value/2(Phase) -> Sum/1
  Discrete 3-phase PLL-Driven Positive-Sequence Fundamental Value/1(Mag) -> Product2/1, Mag_V_V/1
  Discrete 3-phase PLL-Driven Positive-Sequence Fundamental Value2/2(Phase) -> Sum/2
  Sum/1 -> Deg->Rad/1
  Deg->Rad/1 -> Trigonometric Function1/1, Trigonometric Function/1
  Trigonometric Function1/1 -> Product/2
  Trigonometric Function/1 -> Product1/1
  Product/1 -> Gain1/1
  Gain1/1 -> P_W/1
  Product2/1 -> Product/1, Product1/2
  Discrete 3-phase PLL-Driven Positive-Sequence Fundamental Value2/1(Mag) -> Product2/2
  Iabc_A/1 -> Discrete 3-phase PLL-Driven Positive-Sequence Fundamental Value2/3(abc)
  Product1/1 -> Gain2/1
  Gain2/1 -> Q_Var/1

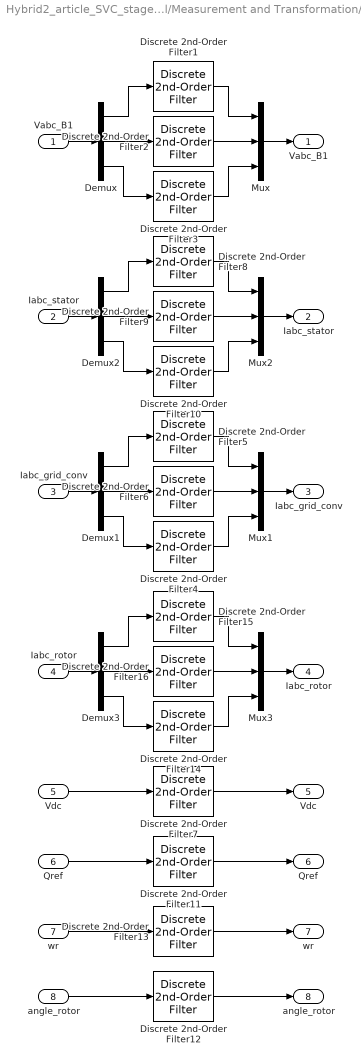
== system Hybrid2_article_SVC_stage1/DFIG Wind Turbine/Control/Measurement and Transformation/Filter ==
  Vabc_B1 : Inport
  Iabc_stator : Inport  Port=2
  Iabc_grid_conv : Inport  Port=3
  Iabc_rotor : Inport  Port=4
  Vdc : Inport  Port=5
  Qref : Inport  Port=6
  wr : Inport  Port=7
  angle_rotor : Inport  Port=8
  Demux{,1..3} (4 alike) : Demux  Outputs=3
      settings: DisplayOption=none
  Discrete 2nd-Order Filter{1..6,8..16} (15 alike) : powerlib_extras/Discrete  Control Blocks/Discrete  2nd-Order Filter  FilterType=Lowpass  Fo=Freq  Zeta=Zeta1  Ts=Ts  Initialize=off  Vac_Init=[0.8 -25 60]  Vdc_Init=-0.4  PlotResponse=off  param1=[1 500 1]
  Discrete 2nd-Order Filter7 : powerlib_extras/Discrete  Control Blocks/Discrete  2nd-Order Filter  FilterType=Lowpass  Fo=Freq  Zeta=Zeta1  Ts=Ts  Initialize=on  Vac_Init=[0.8 -25 60]*0  Vdc_Init=Vdc_nom  PlotResponse=off  param1=[1 500 1]
  Mux{,1..3} (4 alike) : Mux  Inputs=3
  "Vabc_B1 " : Outport  VectorParamsAs1DForOutWhenUnconnected=off
  "Iabc_stator " : Outport  Port=2  VectorParamsAs1DForOutWhenUnconnected=off
  "Iabc_grid_conv " : Outport  Port=3  VectorParamsAs1DForOutWhenUnconnected=off
  "Iabc_rotor " : Outport  Port=4  VectorParamsAs1DForOutWhenUnconnected=off
  "Vdc " : Outport  Port=5  VectorParamsAs1DForOutWhenUnconnected=off
  "Qref " : Outport  Port=6  VectorParamsAs1DForOutWhenUnconnected=off
  "wr " : Outport  Port=7  VectorParamsAs1DForOutWhenUnconnected=off
  "angle_rotor " : Outport  Port=8  VectorParamsAs1DForOutWhenUnconnected=off
  wires:
  Demux/1 -> Discrete 2nd-Order Filter1/1
  Demux/2 -> Discrete 2nd-Order Filter2/1
  Demux/3 -> Discrete 2nd-Order Filter3/1
  Discrete 2nd-Order Filter1/1 -> Mux/1
  Discrete 2nd-Order Filter2/1 -> Mux/2
  Discrete 2nd-Order Filter3/1 -> Mux/3
  Vabc_B1/1 -> Demux/1
  Mux/1 -> "Vabc_B1 "/1
  Demux1/1 -> Discrete 2nd-Order Filter5/1
  Demux1/2 -> Discrete 2nd-Order Filter6/1
  Demux1/3 -> Discrete 2nd-Order Filter4/1
  Discrete 2nd-Order Filter5/1 -> Mux1/1
  Discrete 2nd-Order Filter6/1 -> Mux1/2
  Discrete 2nd-Order Filter4/1 -> Mux1/3
  Iabc_grid_conv/1 -> Demux1/1
  Mux1/1 -> "Iabc_grid_conv "/1
  Vdc/1 -> Discrete 2nd-Order Filter7/1
  Discrete 2nd-Order Filter7/1 -> "Vdc "/1
  Demux2/1 -> Discrete 2nd-Order Filter8/1
  Demux2/2 -> Discrete 2nd-Order Filter9/1
  Demux2/3 -> Discrete 2nd-Order Filter10/1
  Discrete 2nd-Order Filter8/1 -> Mux2/1
  Discrete 2nd-Order Filter9/1 -> Mux2/2
  Discrete 2nd-Order Filter10/1 -> Mux2/3
  Iabc_stator/1 -> Demux2/1
  Mux2/1 -> "Iabc_stator "/1
  wr/1 -> Discrete 2nd-Order Filter13/1
  Discrete 2nd-Order Filter13/1 -> "wr "/1
  Demux3/1 -> Discrete 2nd-Order Filter15/1
  Demux3/2 -> Discrete 2nd-Order Filter16/1
  Demux3/3 -> Discrete 2nd-Order Filter14/1
  Discrete 2nd-Order Filter15/1 -> Mux3/1
  Discrete 2nd-Order Filter16/1 -> Mux3/2
  Discrete 2nd-Order Filter14/1 -> Mux3/3
  Iabc_rotor/1 -> Demux3/1
  Mux3/1 -> "Iabc_rotor "/1
  Qref/1 -> Discrete 2nd-Order Filter11/1
  Discrete 2nd-Order Filter11/1 -> "Qref "/1
  angle_rotor/1 -> Discrete 2nd-Order Filter12/1
  Discrete 2nd-Order Filter12/1 -> "angle_rotor "/1

== system Hybrid2_article_SVC_stage1/DFIG Wind Turbine/Control/Rotor-side Controls/INT ==
  note: INTEGRATOR (Trapezoidal) with External limits & Reset & Hold
  Max : Inport
  Min : Inport  Port=2
  In : Inport  Port=3
  Ki : Inport  Port=4
  Hold : Inport  Port=5
  Reset : Inport  Port=6
  Reset Value : Inport  Port=7
  Gain : Gain  Gain=Ts* 0.5  SaturateOnIntegerOverflow=on  OutDataTypeStr=Inherit: Same as input  ParamDataTypeStr=Inherit: Same as input
  IC = 0 : UnitDelay  SampleTime=Ts  HasFrameUpgradeWarning=on
  IC = i_ic : UnitDelay  SampleTime=Ts  HasFrameUpgradeWarning=on
  Logical Operator4 : Logic  Operator=OR
  MinMax : MinMax  Inputs=2  InputSameDT=on  SaturateOnIntegerOverflow=on
  MinMax1 : MinMax  Function=max  Inputs=2  InputSameDT=on  SaturateOnIntegerOverflow=on
  Product : Product  SaturateOnIntegerOverflow=on  OutDataTypeStr=Inherit: Same as first input
  S6 : Subsystem  mask(Limiter with External Limits){}
      mask Display: disp('      Limiter\n')
  Sum : Sum  InputSameDT=on  SaturateOnIntegerOverflow=on  OutDataTypeStr=Inherit: Same as first input
  Sum1 : Sum  InputSameDT=on  SaturateOnIntegerOverflow=on  OutDataTypeStr=Inherit: Same as first input
  Switch2 : Switch  Threshold=0.5
  Switch3 : Switch  Threshold=0.5
  Switch7 : Switch  Threshold=0.5
  Out : Outport  InitialOutput=0  VectorParamsAs1DForOutWhenUnconnected=off
  wires:
  S6/1("  ") -> IC = i_ic/1, Out/1
  Gain/1 -> Product/1
  Sum1/1 -> Product/2
  Ki/1 -> Gain/1
  IC = 0/1 -> Sum1/2
  In/1 -> IC = 0/1, Sum1/1
  Product/1 -> Sum/1
  Sum/1 -> S6/2(In)
  Hold/1 -> Logical Operator4/1
  Reset/1 -> Switch7/2, Logical Operator4/2
  Logical Operator4/1 -> Switch2/2, Switch3/2
  Switch2/1 -> MinMax/1
  Max/1 -> Switch2/3, MinMax/2
  Reset Value/1 -> Switch7/1
  MinMax/1 -> S6/1(MAX)
  MinMax1/1 -> S6/3(MIN)
  Switch3/1 -> MinMax1/1
  Min/1 -> Switch3/3, MinMax1/2
  IC = i_ic/1 -> Switch7/3
  Switch7/1 -> Switch2/1, Sum/2, Switch3/1

== system Hybrid2_article_SVC_stage1/DFIG Wind Turbine/Control/Rotor-side Controls/Stator flux estimator ==
  note: Quasi steady-state magnitude of flux at generator stator
  Vdqs : Inport
  Idqs : Inport  Port=2
  w_pu : Inport  Port=3
  Abs : Abs  SaturateOnIntegerOverflow=off
  Compare To Constant : simulink/Logic and Bit Operations/Compare To Constant  relop=>=  const=1e-4  OutDataTypeStr=boolean
  Compare To Zero : simulink/Logic and Bit Operations/Compare To Zero  relop=>  OutDataTypeStr=boolean
  Compare To Zero1 : simulink/Logic and Bit Operations/Compare To Zero  relop=>  OutDataTypeStr=boolean
  Constant : Constant  Value=1e-4
  Constant1 : Constant  Value=1e-6
  Constant2 : Constant  Value=1e-6
  Divide1 : Product  Inputs=*/
  Divide2 : Product  Inputs=**
  Divide4 : Product  Inputs=*/
  Divide6 : Product  Inputs=**
  Gain : Gain  Gain=-1
  Lowpass Tau=1/4 cycle : powerlib_extras/Discrete  Control Blocks/Discrete 1st-Order Filter  FilterType=Lowpass  Tc=0.25*(1/Fnom)  Ts=Ts  Initialize=on  Vac_Init=[0.8 -25 60]*0  Vdc_Init=1  PlotResponse=off  param1=[1 500 0.1]
  Math Function1 : Math  Operator=square  SignedPower=on
  Math Function2 : Math  Operator=square  SignedPower=on
  Math Function3 : Math  Operator=sqrt  SignedPower=on
  Rs : Constant  Value=Rs
  Rs2 : Constant  Value=Rs
  Selector1 : Selector  InputPortWidth=2  IndexOptions=Index vector (dialog)  Indices=2  OutputSizes=1
  Selector2 : Selector  InputPortWidth=2  IndexOptions=Index vector (dialog)  Indices=1  OutputSizes=1
  Selector3 : Selector  InputPortWidth=2  IndexOptions=Index vector (dialog)  Indices=2  OutputSizes=1
  Selector4 : Selector  InputPortWidth=2  IndexOptions=Index vector (dialog)  Indices=1  OutputSizes=1
  Sum1 : Sum  Inputs=|++
  Sum2 : Sum  Inputs=|+-
  Sum3 : Sum  Inputs=|+-
  Switch : Switch  Criteria=u2 ~= 0  SaturateOnIntegerOverflow=off  InputSameDT=off
  Switch1 : Switch  Criteria=u2 > Threshold  SaturateOnIntegerOverflow=off  InputSameDT=off
  Switch2 : Switch  Criteria=u2 > Threshold  SaturateOnIntegerOverflow=off  InputSameDT=off
  Mag_Flux : Outport  VectorParamsAs1DForOutWhenUnconnected=off
  wires:
  Math Function2/1 -> Sum1/2
  Divide4/1 -> Math Function2/1  "phi_ds"
  Sum2/1 -> Divide4/1
  Divide2/1 -> Sum2/2  "RsIqs"
  Rs2/1 -> Divide2/2
  Selector3/1 -> Divide2/1  "Iqs"
  Selector1/1 -> Sum2/1  "Vqs"
  Math Function3/1 -> Lowpass Tau=1/4 cycle/1
  Sum1/1 -> Math Function3/1
  Math Function1/1 -> Sum1/1
  Gain/1 -> Abs/1, Switch/3
  Sum3/1 -> Divide1/1
  w_pu/1 -> Compare To Zero1/1, Switch2/1, Gain/1
  Selector4/1 -> Sum3/1  "Vds"
  Vdqs/1 -> Selector1/1, Selector4/1
  Rs/1 -> Divide6/2
  Selector2/1 -> Divide6/1  "ids"
  Divide6/1 -> Sum3/2  "RsIds"
  Idqs/1 -> Selector3/1, Selector2/1
  Lowpass Tau=1/4 cycle/1 -> Mag_Flux/1
  Abs/1 -> Compare To Constant/1
  Compare To Constant/1 -> Switch/2
  Constant/1 -> Switch/1
  Divide1/1 -> Math Function1/1  "phi_qs"
  Constant1/1 -> Switch1/3
  Compare To Zero/1 -> Switch1/2
  Switch/1 -> Switch1/1, Compare To Zero/1
  Switch1/1 -> Divide1/2
  Constant2/1 -> Switch2/3
  Compare To Zero1/1 -> Switch2/2
  Switch2/1 -> Divide4/2

== system Hybrid2_article_SVC_stage1/DFIG Wind Turbine/Control/Speed & Pitch Control/Discrete PI Controller ==
  note: Discrete PID Controller
  note: Pierre Giroux, Gilbert Sybille
      | Power System Simulation Laboratory
      | IREQ, Hydro-Quebc
  Error : Inport
  Discrete-Time Integrator : DiscreteIntegrator  InitialCondition=Init  SampleTime=Ts  LimitOutput=on  UpperSaturationLimit=UpperLimit  LowerSaturationLimit=LowerLimit  ICPrevOutput=DiscIntNeverNeededParam  ICPrevScaledInput=DiscIntNeverNeededParam
  Product1 : Product  RndMeth=Zero
  Product2 : Product  RndMeth=Zero
  Saturation2 : Saturate  UpperLimit=UpperLimit  LowerLimit=LowerLimit
  Step_Ki_speed : Step  Time=999  Before=Ki  After=Ki  SampleTime=Ts
  Step_Kp_speed : Step  Time=999  Before=Kp  After=Kp  SampleTime=Ts
  Sum6 : Sum  InputSameDT=on  SaturateOnIntegerOverflow=on  OutDataTypeStr=Inherit: Same as first input
  Out : Outport  InitialOutput=0  VectorParamsAs1DForOutWhenUnconnected=off
  wires:
  Saturation2/1 -> Out/1
  Discrete-Time Integrator/1 -> Sum6/2
  Product1/1 -> Sum6/1
  Product2/1 -> Discrete-Time Integrator/1
  Sum6/1 -> Saturation2/1
  Error/1 -> Product1/2, Product2/1
  Step_Kp_speed/1 -> Product1/1
  Step_Ki_speed/1 -> Product2/2

== system Hybrid2_article_SVC_stage1/Distribution Statcom1/D_statcom_avg Controller/Controller (sample time=Ts*32)/AC Voltage Regulator ==
  Vac_Ref : Inport
  Mag_V : Inport  Port=2
  Discrete PI Controller : slpidlib/PID Controller  Controller=PI  Form=Parallel  TimeDomain=Discrete-time  UseExternalTs=off  SampleTime=Ts  IntegratorMethod=Forward Euler  FilterMethod=Forward Euler  ControllerParametersSource=internal  P=Kp  I=Ki  UseKiTs=off  D=0  UseExternalDerivativeSource=off  N=100  UseFilter=on  TunerSelectOption=Transfer Function Based (PID Tuner App)  InitialConditionSource=internal  InitialConditionForIntegrator=0  InitialConditionForFilter=0  DifferentiatorICPrevScaledInput=0  ExternalReset=none  TrackingMode=off  Kt=1  LimitOutput=on  SatLimitsSource=internal  UpperSaturationLimit=1  LowerSaturationLimit=-1  LinearizeAsGain=off  AntiWindupMode=clamping  Kb=1  LimitIntegrator=off  UpperIntegratorSaturationLimit=inf  LowerIntegratorSaturationLimit=-inf  POutMin=[]  POutMax=[]  IOutMin=[]  IOutMax=[]  DOutMin=[]  DOutMax=[]  NOutMin=[]  NOutMax=[]  SumOutMin=[]  SumOutMax=[]  SaturationOutMin=[]  SaturationOutMax=[]  PParamMin=[]  PParamMax=[]  IParamMin=[]  IParamMax=[]  DParamMin=[]  DParamMax=[]  NParamMin=[]  NParamMax=[]  KbParamMin=[]  KbParamMax=[]  KtParamMin=[]  KtParamMax=[]  KbOutMin=[]  KbOutMax=[]  KtOutMin=[]  KtOutMax=[]  IntegratorOutMin=[]  IntegratorOutMax=[]  FilterOutMin=[]  FilterOutMax=[]  SumI1OutMin=[]  SumI1OutMax=[]  SumI2OutMin=[]  SumI2OutMax=[]  SumI3OutMin=[]  SumI3OutMax=[]  SumI4OutMin=[]  SumI4OutMax=[]  SumDOutMin=[]  SumDOutMax=[]  DifferentiatorOutMin=[]  DifferentiatorOutMax=[]  FilterDiffOutCoefMin=[]  FilterDiffOutCoefMax=[]  ReciprocalOutMin=[]  ReciprocalOutMax=[]  SumDenOutMin=[]  SumDenOutMax=[]  SumNumOutMin=[]  SumNumOutMax=[]  DivideOutMin=[]  DivideOutMax=[]  UdiffTsProdOutMin=[]  UdiffTsProdOutMax=[]  NTsProdOutMin=[]  NTsProdOutMax=[]  UintegralTsProdOutMin=[]  UintegralTsProdOutMax=[]  UngainTsProdOutMin=[]  UngainTsProdOutMax=[]  ClampingZeroOutDataTypeStr=Inherit: Inherit via back propagation  ClampingZeroOutMin=[]  ClampingZeroOutMax=[]  FilterDenConstantOutDataTypeStr=Inherit: Inherit via back propagation  FilterDenConstantOutMin=[]  FilterDenConstantOutMax=[]  PCopyOutDataTypeStr=Inherit: Inherit via back propagation  PCopyOutMin=[]  PCopyOutMax=[]  NCopyOutDataTypeStr=Inherit: Inherit via back propagation  NCopyOutMin=[]  NCopyOutMax=[]  IntegratorContinuousStateAttributes=''  IntegratorStateMustResolveToSignalObject=off  IntegratorRTWStateStorageClass=Auto  FilterContinuousStateAttributes=''  FilterStateMustResolveToSignalObject=off  FilterRTWStateStorageClass=Auto  ParallelPVariant=InternalParameters  IdealPVariant=Disabled  IVariant=InternalParameters  DVariant=Disabled  IntegratorVariant=Discrete  SatVariant=Enabled  AWVariant=DiscClampingParallel  PCopyVariant=Disabled  TRVariant=Disabled  FdbkBlocksVariant=Forward  IdealPFdbkVariant=Disabled  SatFdbkVariant=Disabled  DerivativeFilterVariant=Disabled  NVariant=Disabled  NCopyVariant=Disabled_SignalSpec  FilterICVariant=Disabled  IntegratorICVariant=InternalICs  ExternalResetVariant=Disabled  TRSumVariant=Passthrough  SumFdbkVariant=Disabled  SumVariant=Sum_PI  TsampFilterVariant=InternalTs  TsampNgainVariant=Passthrough  TsampIntegralVariant=Disabled_SignalSpec  ExternalSaturationOutDataTypeStr=Inherit: Same as second input  DerivativeSourceVariant=Disabled  PreIntVariant=InternalPreInt
      settings: AttributesFormatString=P = %<P>\nI = %<I>
  Sum : Sum  Inputs=|+-  InputSameDT=on  SaturateOnIntegerOverflow=on  OutDataTypeStr=Inherit: Same as first input
  Iq_Ref : Outport  InitialOutput=0  VectorParamsAs1DForOutWhenUnconnected=off
  wires:
  Vac_Ref/1 -> Sum/1
  Mag_V/1 -> Sum/2
  Sum/1 -> Discrete PI Controller/1
  Discrete PI Controller/1 -> Iq_Ref/1
